simulink model "DCDC_Converter"  (R2024a)
settings: Solver=VariableStepAuto  StartTime=0.0  StopTime=20  RelTol=1e-3
InitFcn:
  |  if any(exist('rtifpga_mdlclblib', 'file') ~= 0), rtifpga_mdlclblib('Init', bdroot); end,
  | Ts  = 1e-7;
  | T_PWM = 1e-4;
  | T_MPPT = 1e-2;
  | Ts  = T_PWM / 200;
  | 
  | Vpeak = 170;
  | Vnom = Vpeak*sqrt(3)/sqrt(2);
  | Fnom = 60;
  | w_rad  = 2*pi*Fnom;
  | 
  | Vdc2 = 300;
  | 
  | % LC filter for DG1
  | L11 = 5e-03;
  | Cf1 = 30e-06;
  | Rc1 = 0.5;           % Damping series-resistor
  | RL1 = 0.9;        % Inductor ESR
  | L22=1e-12;
  | % LC filter for DG2
  | L12 = 5e-03;
  | Cf2 = 10e-06;
  | Rc2 = 0.5;           % Damping series-resistor
  | RL2 = 0.9;        % Inductor ESR
  | 
  | Pnom = 1000;
libraries: dspfdesign x3, spsSeriesRLCBranchLib x3, spsDiodeLib x1, spsMosfetLib x1, spsPVArrayLib x1, simulink x1, spsVoltageMeasurementLib x1, sps_lib x1
settings Model: SimulationMode=accelerator  Creator=calum  LastModifiedBy=nicho

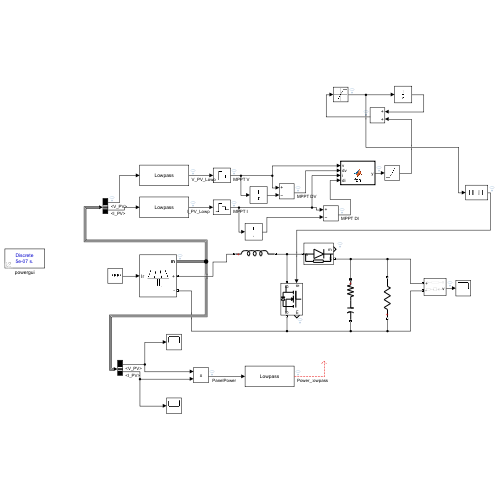
[thumbnail: Simulink's stored preview of the top-level diagram]
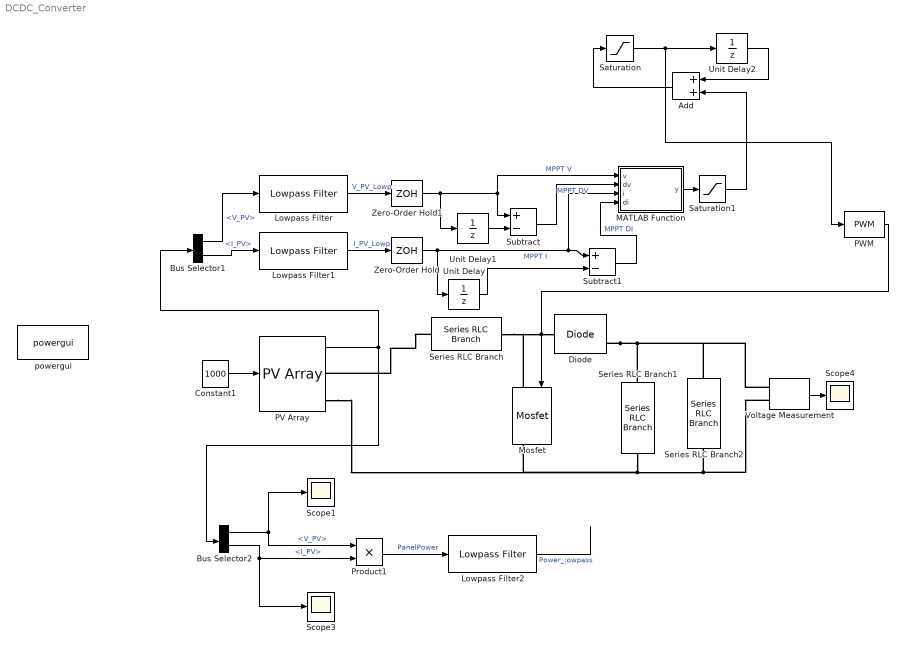
== system DCDC_Converter ==
  Add : Sum
  Bus Selector1 : BusSelector  OutputSignals=V_PV,I_PV
  Bus Selector2 : BusSelector  OutputSignals=V_PV,I_PV
  Constant1 : Constant  Value=1000
  Diode : spsDiodeLib/Diode  Ron=0.001  Lon=0  Vf=0.8  IC=0  UseSnubber=0  Rs=5e6  Cs=250e-9  Measurements=on
  Lowpass Filter : dspfdesign/Lowpass Filter  FilterType=FIR  DesignForMinimumOrder=on  FilterOrder=5  PassbandFrequency=4/T_MPPT  StopbandFrequency=1/T_PWM  PassbandRipple=0.01  StopbandAttenuation=80  SampleRate=44100  SimulateUsing=Code generation  roundingMode=Floor  coeffsDataTypeStr=fixdt(1,16)
  Lowpass Filter1 : dspfdesign/Lowpass Filter  FilterType=FIR  DesignForMinimumOrder=on  FilterOrder=5  PassbandFrequency=4/T_MPPT  StopbandFrequency=1/T_PWM  PassbandRipple=0.01  StopbandAttenuation=80  SampleRate=44100  SimulateUsing=Code generation  roundingMode=Floor  coeffsDataTypeStr=fixdt(1,16)
  Lowpass Filter2 : dspfdesign/Lowpass Filter  FilterType=FIR  DesignForMinimumOrder=on  FilterOrder=5  PassbandFrequency=10/T_MPPT  StopbandFrequency=1/T_PWM  PassbandRipple=0.01  StopbandAttenuation=80  SampleRate=44100  SimulateUsing=Code generation  roundingMode=Floor  coeffsDataTypeStr=fixdt(1,16)
  MATLAB Function : MATLAB Function  TreatAsAtomicUnit=on
  Mosfet : spsMosfetLib/Mosfet  Ron=0.001  Lon=0  Rd=0.01  Vfd=0  IC=0  Rs=1e9  Cs=inf  Measurements=on
  PV Array : spsPVArrayLib/PV Array  Npar=10  Nser=2  PlotType=array @ 1000 W/m2 & specified temperatures  S_vec="[ 1000  500  100 ]"  Temp_C_vec=[ 45 20 ]  ModuleName=A10Green Technology A10J-S72-175  PlotWhenSelected=off  Pm=175.0914  Ncell=72  Voc=43.99  Isc=5.17  Vm=36.63  Im=4.78  beta_Voc_pc=-0.3616  alpha_Isc_pc=0.041509  beta_Voc=-0.15907  alpha_Isc=0.002146  IL=5.178  I0=1.7842e-10  nI=0.98852  Rsh=249.6758  Rs=0.38412  RobustModel=on  RobustCellTemperature=20  BAL=on  Tc=1e-6  Tfilter=5e-5
  PWM : simulink/Discontinuities/PWM  DisableCoverage=on  Period=.0001  InitialDelay=0  DisallowZeroDutyCycle=off  RunAtFixedTimeIntervals=off  SampleTime=0.1
  Product1 : Product
  Saturation : Saturate  UpperLimit=.999  LowerLimit=0.001
  Saturation1 : Saturate  UpperLimit=.005  LowerLimit=-.005
  Scope1 : Scope
  Scope3 : Scope
  Scope4 : Scope
  Series RLC Branch : spsSeriesRLCBranchLib/Series RLC Branch  LConnTagsString=__new0  RConnTagsString=__new0  BranchType=L  Resistance=1  Inductance=2e-3  SetiL0=off  InitialCurrent=0  Capacitance=0  Setx0=off  InitialVoltage=0  Measurements=None
  Series RLC Branch1 : spsSeriesRLCBranchLib/Series RLC Branch  LConnTagsString=__new0  RConnTagsString=__new0  BranchType=RC  Resistance=.001  Inductance=1e-3  SetiL0=off  InitialCurrent=0  Capacitance=470e-6  Setx0=off  InitialVoltage=0  Measurements=None
  Series RLC Branch2 : spsSeriesRLCBranchLib/Series RLC Branch  LConnTagsString=__new0  RConnTagsString=__new0  BranchType=R  Resistance=50  Inductance=1e-3  SetiL0=off  InitialCurrent=0  Capacitance=1e-2  Setx0=off  InitialVoltage=0  Measurements=None
  Subtract : Sum  Inputs=+-
  Subtract1 : Sum  Inputs=+-
  Unit Delay : UnitDelay  SampleTime=T_MPPT  HasFrameUpgradeWarning=on
  Unit Delay1 : UnitDelay  SampleTime=T_MPPT  HasFrameUpgradeWarning=on
  Unit Delay2 : UnitDelay  InitialCondition=0.5  SampleTime=T_MPPT  HasFrameUpgradeWarning=on
  Voltage Measurement : spsVoltageMeasurementLib/Voltage Measurement  PhasorSimulation=off  OutputType=Complex  PSBequivalent=0
  Zero-Order Hold : ZeroOrderHold  SampleTime=T_MPPT
  Zero-Order Hold1 : ZeroOrderHold  SampleTime=T_MPPT
  powergui : sps_lib/powergui  Priority=1  SimulationMode=Discrete  SampleTime=Ts  frequency=60  Iterations=50  frequencyindice=0  Pbase=100e6  ErrMax=1e-4  UnitsV=kV  UnitsW=MW  buscounter=0  FunctionMessages=off  echomessages=off  EnableUseOfTLC=off  CurrentSourceSwitches=off  DisableSnubberDevices=off  DisableRonSwitches=off  DisableVfSwitches=off  DisplayEquations=off  AutomaticDiscreteSolvers=off  SolverType=Tustin/Backward Euler (TBE)  Interpol=off  ExternalGateDelay=off  methode=off  Ts=100  x0status=blocks  SPID=on  SwTol=0  HookPort=off  NonlinearTolerance=1e-4  nMaxIteration=100  ContinueOnMaxIteration=off  RestoreLinks=warning  ResistiveCurrentMeasurement=off  Frange=[0:2:500]  Ylog=off  Xlog=on  ShowGrid=off  save=off  variable=ZData  structure=0  ZoomFFT=off  StartTime=0.0  cycles=1  DisplayStyle=1  fundamental=60  FreqAxis=off  MaxFrequency=1000  frequencyindicesteady=1  RmsSteady=1  display=off
  wires:
  Voltage Measurement/1 -> Scope4/1
  PWM/1 -> Mosfet/1
  Product1/1 -> Lowpass Filter2/1  "PanelPower"
  Bus Selector2/1 -> Scope1/1, Product1/1  "<V_PV>"
  Bus Selector2/2 -> Scope3/1, Product1/2  "<I_PV>"
  Constant1/1 -> PV Array/1
  PV Array/1 -> Bus Selector1/1, Bus Selector2/1
  Bus Selector1/1 -> Lowpass Filter/1  "<V_PV>"
  Bus Selector1/2 -> Lowpass Filter1/1  "<I_PV>"
  Lowpass Filter/1 -> Zero-Order Hold1/1  "V_PV_Lowp"
  Lowpass Filter1/1 -> Zero-Order Hold/1  "I_PV_Lowp"
  Zero-Order Hold/1 -> Unit Delay/1, Subtract1/1, MATLAB Function/3(i)  "MPPT I"
  Zero-Order Hold1/1 -> MATLAB Function/1(v), Subtract/1, Unit Delay1/1  "MPPT V"
  Add/1 -> Saturation/1
  Saturation/1 -> Unit Delay2/1, PWM/1
  Unit Delay1/1 -> Subtract/2
  Subtract/1 -> MATLAB Function/2(dv)  "MPPT DV"
  Subtract1/1 -> MATLAB Function/4(di)  "MPPT DI"
  Unit Delay/1 -> Subtract1/2
  Unit Delay2/1 -> Add/1
  MATLAB Function/1(y) -> Saturation1/1
  Saturation1/1 -> Add/2
  Lowpass Filter2/1 -> ?  "Power_:owpass"
  connections:
  Diode/RConn1 -- Series RLC Branch1/LConn1 -- Series RLC Branch2/RConn1 -- Voltage Measurement/LConn1
  Voltage Measurement/LConn2 -- PV Array/RConn2 -- Mosfet/RConn1 -- Series RLC Branch1/RConn1 -- Series RLC Branch2/LConn1
  Series RLC Branch/LConn1 -- PV Array/RConn1
  Diode/LConn1 -- Series RLC Branch/RConn1 -- Mosfet/LConn1

== matlab function DCDC_Converter/MATLAB Function ==
  data: v input; y output; dv input; i input; di input
function y = fcn(v, dv, i, di)


if(dv == 0)
    % if there is no dv, return a correction proportional to
    % change in current (or zero, if current is zero)
    y = di / 40000;
    return
end

y = -(i + di / dv * v)/40000;
return
